simulink model "Model_tn84"  (R2020b)
settings: Solver=VariableStepAuto  StartTime=0.0  StopTime=120  RelTol=1e-3
libraries: SignalEditorBlockLib x1
settings Model: Creator=Stend  LastModifiedBy=Stend

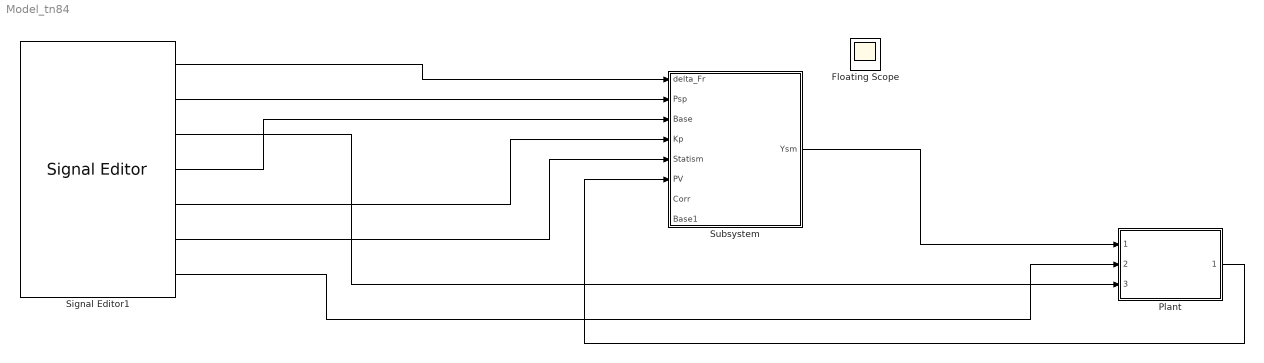
== system Model_tn84 ==
  Floating Scope : Scope
      settings: Floating=on
  Plant : Subsystem  ReferencedSubsystem=Plant
  Signal Editor1 : SignalEditorBlockLib/Signal Editor  FileName=Psp_deltaFr.mat  ActiveScenario=Scenario1  ActiveSignal=delta_Fr  IsBus=off  OutputBusObjectStr=Bus: BusObject  SampleTime=0  Interpolate=off  ZeroCross=off  OutputAfterFinalValue=Setting to zero  Unit=inherit  PreserveSignalName=on
  Subsystem : Subsystem
  wires:
  Signal Editor1/7 -> Plant/2
  Signal Editor1/3 -> Plant/3
  Signal Editor1/1 -> Subsystem/1(delta_Fr)
  Signal Editor1/2 -> Subsystem/2(Psp)
  Signal Editor1/4 -> Subsystem/3(Base)
  Signal Editor1/5 -> Subsystem/4(Kp)
  Signal Editor1/6 -> Subsystem/5(Statism)
  Plant/1 -> Subsystem/6(PV)
  Subsystem/1(Ysm) -> Plant/1

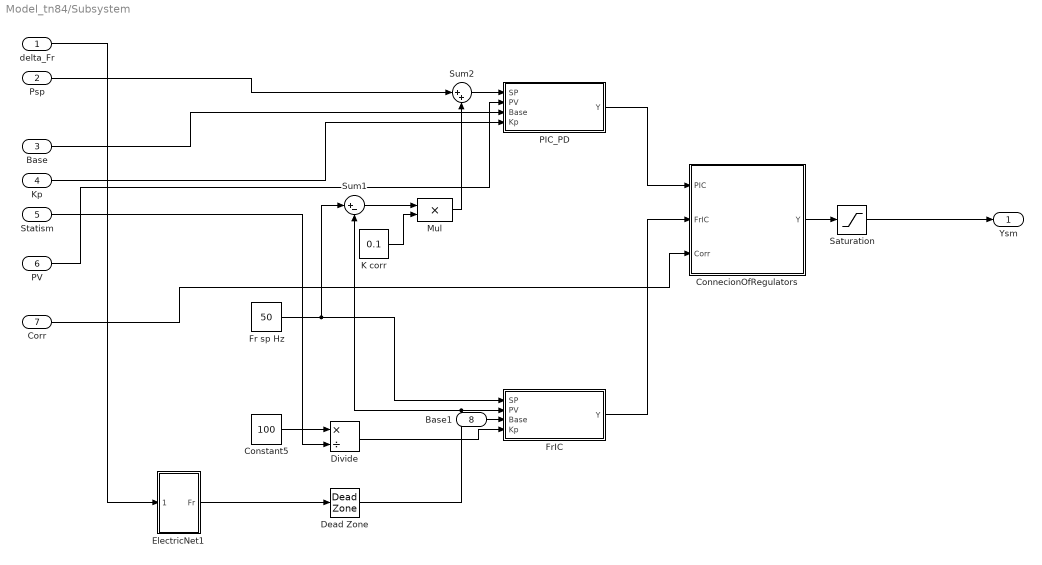
== system Model_tn84/Subsystem ==
  delta_Fr : Inport
  Psp : Inport  Port=2
  Base : Inport  Port=3
  Kp : Inport  Port=4
  Statism : Inport  Port=5
  PV : Inport  Port=6
  Corr : Inport  Port=7
  Base1 : Inport  Port=8
  ConnecionOfRegulators : Subsystem
  Constant5 : Constant  Value=100
  Dead Zone : DeadZone  LowerValue=-0.02  UpperValue=0.02  SaturateOnIntegerOverflow=on
  Divide : Product  Inputs=*/
  ElectricNet1 : Subsystem
  Fr sp Hz : Constant  Value=50
  FrIC : Subsystem  TreatAsAtomicUnit=on
  K corr : Constant  Value=0.1
  Mul : Product  InputSameDT=on  SaturateOnIntegerOverflow=on  OutDataTypeStr=Inherit: Same as first input
  PIC_PD : Subsystem  TreatAsAtomicUnit=on
  Saturation : Saturate  UpperLimit=100  LowerLimit=0
  Sum1 : Sum  Inputs=|+-  InputSameDT=on  SaturateOnIntegerOverflow=on  OutDataTypeStr=Inherit: Same as first input
  Sum2 : Sum  Inputs=|++  InputSameDT=on  SaturateOnIntegerOverflow=on  OutDataTypeStr=Inherit: Same as first input
  Ysm : Outport
  wires:
  FrIC/1(Y) -> ConnecionOfRegulators/2(FrIC)
  Mul/1 -> Sum2/2
  Dead Zone/1 -> FrIC/2(PV), Sum1/2
  Fr sp Hz/1 -> FrIC/1(SP), Sum1/1
  Kp/1 -> PIC_PD/4(Kp)
  K corr/1 -> Mul/2
  Divide/1 -> FrIC/4(Kp)
  Sum2/1 -> PIC_PD/1(SP)
  Saturation/1 -> Ysm/1
  ElectricNet1/1(Fr) -> Dead Zone/1
  Sum1/1 -> Mul/1
  Constant5/1 -> Divide/1
  Corr/1 -> ConnecionOfRegulators/3(Corr)
  ConnecionOfRegulators/1(Y) -> Saturation/1
  PIC_PD/1(Y) -> ConnecionOfRegulators/1(PIC)
  PV/1 -> PIC_PD/2(PV)
  Statism/1 -> Divide/2
  Base1/1 -> FrIC/3(Base)
  delta_Fr/1 -> ElectricNet1/1(delta_Fr)
  Psp/1 -> Sum2/1
  Base/1 -> PIC_PD/3(Base)

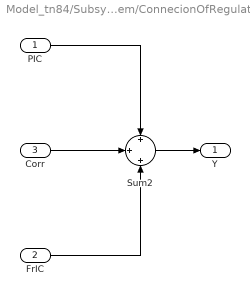
== system Model_tn84/Subsystem/ConnecionOfRegulators ==
  PIC : Inport
  FrIC : Inport  Port=2
  Corr : Inport  Port=3
  Sum2 : Sum  Inputs=+|+|+  InputSameDT=on  SaturateOnIntegerOverflow=on  OutDataTypeStr=Inherit: Same as first input
  Y : Outport
  wires:
  PIC/1 -> Sum2/1
  Sum2/1 -> Y/1
  FrIC/1 -> Sum2/3
  Corr/1 -> Sum2/2

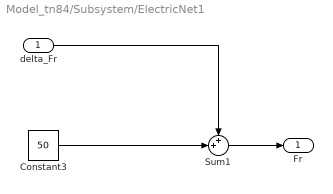
== system Model_tn84/Subsystem/ElectricNet1 ==
  delta_Fr : Inport
  Constant3 : Constant  Value=50
  Sum1 : Sum  Inputs=++|  InputSameDT=on  SaturateOnIntegerOverflow=on  OutDataTypeStr=Inherit: Same as first input
  Fr : Outport
  wires:
  Sum1/1 -> Fr/1
  Constant3/1 -> Sum1/2
  delta_Fr/1 -> Sum1/1

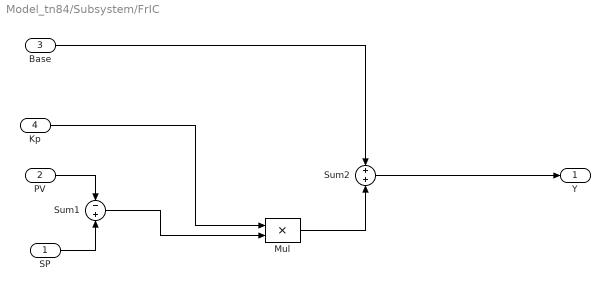
== system Model_tn84/Subsystem/FrIC ==
  SP : Inport
  PV : Inport  Port=2
  Base : Inport  Port=3
  Kp : Inport  Port=4
  Mul : Product  InputSameDT=on  SaturateOnIntegerOverflow=on  OutDataTypeStr=Inherit: Same as first input
  Sum1 : Sum  Inputs=-+  InputSameDT=on  SaturateOnIntegerOverflow=on  OutDataTypeStr=Inherit: Same as first input
  Sum2 : Sum  InputSameDT=on  SaturateOnIntegerOverflow=on  OutDataTypeStr=Inherit: Same as first input
  Y : Outport  OutputWhenDisabled=reset  InitialOutput=0  VectorParamsAs1DForOutWhenUnconnected=off
  wires:
  Kp/1 -> Mul/1
  Base/1 -> Sum2/1
  Sum2/1 -> Y/1
  PV/1 -> Sum1/1
  SP/1 -> Sum1/2
  Sum1/1 -> Mul/2
  Mul/1 -> Sum2/2

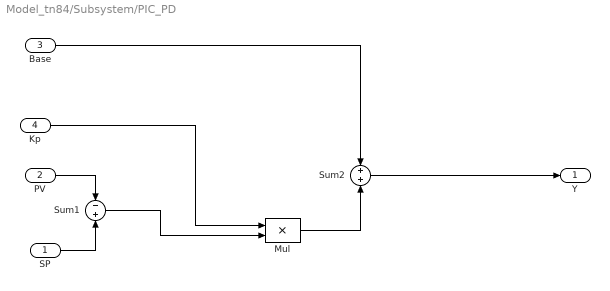
== system Model_tn84/Subsystem/PIC_PD ==
  SP : Inport
  PV : Inport  Port=2
  Base : Inport  Port=3
  Kp : Inport  Port=4
  Mul : Product  InputSameDT=on  SaturateOnIntegerOverflow=on  OutDataTypeStr=Inherit: Same as first input
  Sum1 : Sum  Inputs=-+  InputSameDT=on  SaturateOnIntegerOverflow=on  OutDataTypeStr=Inherit: Same as first input
  Sum2 : Sum  InputSameDT=on  SaturateOnIntegerOverflow=on  OutDataTypeStr=Inherit: Same as first input
  Y : Outport  OutputWhenDisabled=reset  InitialOutput=0  VectorParamsAs1DForOutWhenUnconnected=off
  wires:
  Kp/1 -> Mul/1
  Base/1 -> Sum2/1
  Sum2/1 -> Y/1
  PV/1 -> Sum1/1
  SP/1 -> Sum1/2
  Sum1/1 -> Mul/2
  Mul/1 -> Sum2/2
